simulink model "ltrdemo1"  (Simulink 4.2)
settings: Solver=ode23  SolverMode=SingleTasking  StartTime=0.0  StopTime=200  MaxStep=0.1  RelTol=1e-3  AbsTol=1e-6
PreLoadFcn:
  | ltrdata1
values from neighbouring files (symbols this model uses):
  a = mklti(a,b1,b2,c1,c2,d11,d12,d21,d22,Ts,'tss')    [augss.m]    (also in bilin.m = -xx(1,2); des2ss.m = ue'*a*ve; fitgain.m = ss_; h2data.m = [  -1.0285    0.9853   -0.9413    0.0927)
  b = -xx(1,1)    [bilin.m]    (also in clxbode.m = b(:,iu); des2ss.m = ue'*b; dfreqrc.m = p'*b; h2data.m = [         0)
  c = xx(1,3)    [bilin.m]    (also in des2ss.m = c*ve; dfreqrc.m = c*p; h2data.m = [  -1.7786    1.1390         0   -1.0294]; hinfdata.m = [  -1.7786    1.1390         0   -1.0294])
  d = xx(1,4)    [bilin.m]    (also in clxbode.m = d(:,iu); cschur.m = abs(diag(t)); h2data.m = 0; hinfdata.m = 0)
settings Model: Creator=eyarrow  LastModifiedBy=eyarrow  ExternalInput=[]  SaveTime=off  SaveOutput=off  InitialState=[]  LimitDataPoints=off  IntegerOverflowMsg=none  RTWTemplateMakefile=grt_unix.tmf  ExtModeMexFile=ext_comm.c  ExtModeTrigMode=oneshot  ExtModeArmWhenConnect=off

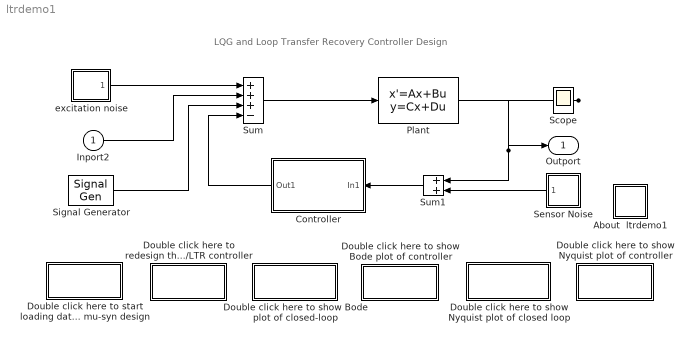
== system ltrdemo1 ==
  note: LQG and Loop Transfer Recovery Controller Design
  Inport2 : Inport  Port=1  LatchInput=off
  About  ltrdemo1 : Subsystem
      settings: OpenFcn=clc; more(24); help ltrdata1; more off;  RTWFcnNameOpts=Auto  RTWFileNameOpts=Auto
      mask Display: disp('?')
  Controller : Subsystem  Orientation=left  mask{@1=ae, @2=be, @3=ce, @4=de}
      mask prompts: @1 "Controller Matrix A:"; @2 "Controller Matrix B:"; @3 "Controller Matrix C:"; @4 "Controller Matrix D:"
      mask help:
      | LTR controller.
      | (Requires Control Toolbox and RCT)
      mask init:
      | ae=@1; be=@2; ce=@3; de=@4;
      settings: RTWFcnNameOpts=Auto  RTWFileNameOpts=Auto
      mask Help: LTR controller design. Mask and unmask this block to see how it works.
      mask Display: disp('LQG/LTR')
  Double click here to redesign the LQG/LTR controller : Subsystem
      settings: OpenFcn=if ~exist('ltry'),fprintf('\nMust be licensed for RCT Toolbox\n'), else, fprintf('\nCtrl_C to abort RCT Calculation\n\n'); ltrdes1; end  RTWFcnNameOpts=Auto  RTWFileNameOpts=Auto
      mask Display: disp('Re-design')
  Double click here to show Bode plot of closed-loop : Subsystem
      settings: OpenFcn=if ~exist('ae'),fprintf('\nMust Load Data & Design First\n'),else [x,y,z,w]=feedback(a,b,c,d,ae,be,ce,de,-1); [x,y,w]=bode(x,y,z,w); clf; subplot(211); loglog(w,x(:,1)); subplot(212); semilogx(w,y(:,1)); subplot(111);end  RTWFcnNameOpts=Auto  RTWFileNameOpts=Auto
      mask Display: disp('Closed-Loop\nBode Plot')
  Double click here to show Bode plot of controller : Subsystem
      settings: OpenFcn="if ~exist('ae'),fprintf('\\nMust Load Data & Design First\\n'),else  [x,y,w]=bode(ae,be,ce,de); clf; subplot(211); loglog(w,x(:,1)); subplot(212); semilogx(w,y(:,1)); subplot(111);end"  RTWFcnNameOpts=Auto  RTWFileNameOpts=Auto
      mask Display: disp('Controller\nBode Plot')
  Double click here to show Nyquist plot of closed loop : Subsystem
      settings: OpenFcn=if ~exist('ae'), fprintf('\nMust Load Data & Desgin First\n'), else,[x,y,z,w]=feedback(a,b,c,d,ae,be,ce,de,-1); clf, nyquist(x,y,z,w); end  RTWFcnNameOpts=Auto  RTWFileNameOpts=Auto
      mask Display: disp('Closed-Loop\nNyquist')
  Double click here to show Nyquist plot of controller : Subsystem
      settings: OpenFcn=if ~exist('ae'), fprintf('\nMust Load Data & Desgin First\n'), else,clf; nyquist(ae,be,ce,de), end  RTWFcnNameOpts=Auto  RTWFileNameOpts=Auto
      mask Display: disp('Controller\nNyquist')
  Double click here to start loading data and mu-syn design : Subsystem
      settings: OpenFcn=if ~exist('ltry'),fprintf('\nMust be licensed for RCT Toolbox\n'), else, ltrdata1; end  RTWFcnNameOpts=Auto  RTWFileNameOpts=Auto
      mask Display: disp('Re-Load\nData')
  Plant : StateSpace  A=a  B=b  C=c  D=d  X0=0  AbsoluteTolerance=auto  Realization=auto
  Scope : Scope
      settings: TickLabels=on  TimeRange=10.000000  YMin=-5  YMax=5  SaveToWorkspace=off  SaveName=ScopeData  DataFormat=Array  LimitDataPoints=on  MaxDataPoints=5000
  Sensor Noise : Subsystem  Orientation=left  mask{@1=0.01, @2=0.11, @3=23341}
      mask prompts: @1 "Noise Variance:"; @2 "Sample Time:"; @3 "Seed"
      mask help:
      | White noise for continuous (s-domain) systems.
      | Band-limited using zero-order-hold.
      mask init:
      | Cov = @1; Ts = @2; seed = @3;
      settings: RTWFcnNameOpts=Auto  RTWFileNameOpts=Auto
      mask Help: Implemented using white noise into Zero Order Hold block. For faster simulation set sample time to highest value possible but in accordance with the fastest dynamics of system.
      mask Display: plot(1:20,rand(1,20))
  Signal Generator : SignalGenerator  WaveForm=sine  Amplitude=1  Frequency=1  Units=Hertz
  Sum : Sum  Inputs=+++-  SaturateOnIntegerOverflow=on
  Sum1 : Sum  Orientation=left  Inputs=++  SaturateOnIntegerOverflow=on
  excitation noise : Subsystem  mask{@1=0.1, @2=1, @3=68932234}
      mask prompts: @1 "Noise Power:"; @2 "Sample Time:"; @3 "Seed"
      mask help:
      | White noise for continuous (s-domain) systems.
      | Band-limited using zero-order-hold.
      mask init:
      | Cov = @1; Ts = @2; seed = @3; r = rand(1,12); r2 = [r(1),r;r,r(12)]; t =[1:13;1:13];
      settings: RTWFcnNameOpts=Auto  RTWFileNameOpts=Auto
      mask Help: Implemented using white noise into Zero-Order Hold block. The seed and power can be vectors of the same length to produce a vector of white noise sources. For faster simulation, set sample time to the highest value possible but in accordance with the fastest dynamics of system.
      mask Display: plot(t(:),r2(:))
  Outport : Outport  Port=1  InitialOutput=0
  wires:
  Sensor Noise/1(out_1) -> Sum1/2
  excitation noise/1(Out_1) -> Sum/1
  Controller/1(Out1) -> Sum/4
  Sum1/1 -> Controller/1(In1)
  Signal Generator/1 -> Sum/3
  Inport2/1 -> Sum/2
  Sum/1 -> Plant/1
  Plant/1 -> Sum1/1, Outport/1, Scope/1

== system ltrdemo1/About  ltrdemo1 ==

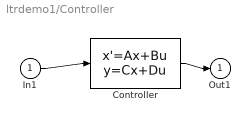
== system ltrdemo1/Controller ==
  In1 : Inport  Port=1  LatchInput=off
  Controller : StateSpace  A=ae  B=be  C=ce  D=de  X0=0  AbsoluteTolerance=auto  Realization=auto
  Out1 : Outport  Port=1  InitialOutput=0
  wires:
  In1/1 -> Controller/1
  Controller/1 -> Out1/1

== system ltrdemo1/Double click here to redesign the LQG/LTR controller ==

== system ltrdemo1/Double click here to show Bode plot of closed-loop ==

== system ltrdemo1/Double click here to show Bode plot of controller ==

== system ltrdemo1/Double click here to show Nyquist plot of closed loop ==

== system ltrdemo1/Double click here to show Nyquist plot of controller ==

== system ltrdemo1/Double click here to start loading data and mu-syn design ==

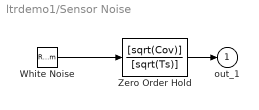
== system ltrdemo1/Sensor Noise ==
  White Noise : RandomNumber  Mean=0  Variance=1  Seed=seed  SampleTime=Ts
  Zero Order Hold : DiscreteTransferFcn  Numerator=[sqrt(Cov)]  Denominator=[sqrt(Ts)]  SampleTime=Ts  Realization=auto
      settings: RTWStateStorageClass=Auto
  out_1 : Outport  Port=1  InitialOutput=0
  wires:
  Zero Order Hold/1 -> out_1/1
  White Noise/1 -> Zero Order Hold/1

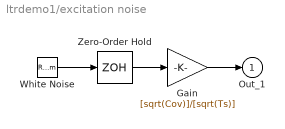
== system ltrdemo1/excitation noise ==
  Gain : Gain  Gain=[sqrt(Cov)]/[sqrt(Ts)]  Multiplication=Element-wise(K.*u)  SaturateOnIntegerOverflow=on
  White Noise : RandomNumber  Mean=0  Variance=1  Seed=seed  SampleTime=Ts
  Zero-Order Hold : ZeroOrderHold  SampleTime=Ts
  Out_1 : Outport  Port=1  InitialOutput=0
  wires:
  White Noise/1 -> Zero-Order Hold/1
  Gain/1 -> Out_1/1
  Zero-Order Hold/1 -> Gain/1
